simulink model "TST_BattU_VD"  (R2016b)
settings: Solver=FixedStepDiscrete  StartTime=0.0  StopTime=simTime  FixedStep=sampleTime  RelTol=1e-3
values from neighbouring files (symbols this model uses):
  testCase = 1    [initTST_BattU_VD_001.m]    (also in initTST_BattU_VD_002.m = 2; initTST_BattU_VD_003.m = 3; initTST_BattU_VD_004.m = 4; initTST_BattU_VD_005.m = 5)
libraries: simulink x21, UnitTest_Lib x15
settings Model: Creator=zhengjinyan  LastModifiedBy=zhengjinyan
settings DebuggingCC: SignalRangeChecking=error

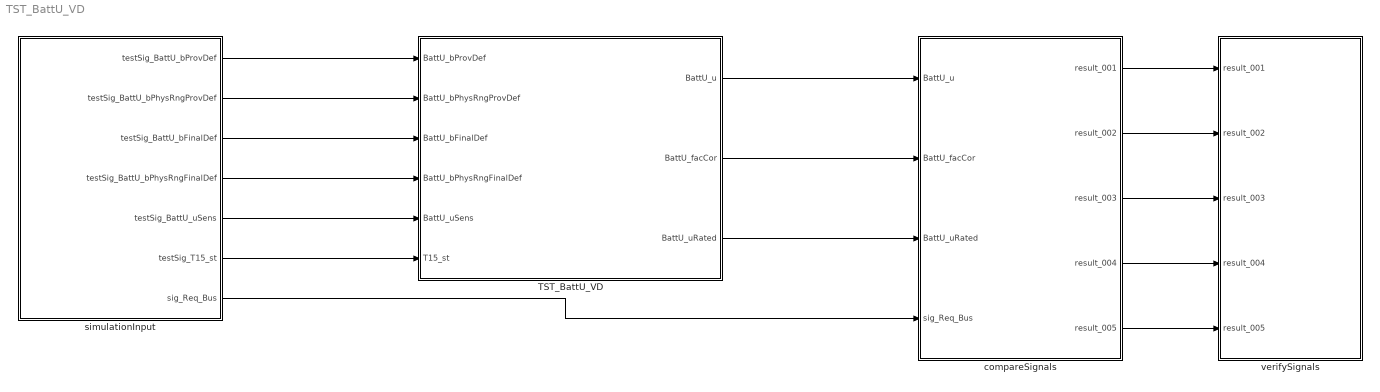
== system TST_BattU_VD ==
  TST_BattU_VD : Subsystem
  compareSignals : Subsystem
  simulationInput : Subsystem
  verifySignals : Subsystem
  wires:
  simulationInput/1(testSig_BattU_bProvDef) -> TST_BattU_VD/1(BattU_bProvDef)
  simulationInput/2(testSig_BattU_bPhysRngProvDef) -> TST_BattU_VD/2(BattU_bPhysRngProvDef)
  simulationInput/3(testSig_BattU_bFinalDef) -> TST_BattU_VD/3(BattU_bFinalDef)
  simulationInput/4(testSig_BattU_bPhysRngFinalDef) -> TST_BattU_VD/4(BattU_bPhysRngFinalDef)
  simulationInput/5(testSig_BattU_uSens) -> TST_BattU_VD/5(BattU_uSens)
  simulationInput/6(testSig_T15_st) -> TST_BattU_VD/6(T15_st)
  TST_BattU_VD/1(BattU_u) -> compareSignals/1(BattU_u)
  TST_BattU_VD/2(BattU_facCor) -> compareSignals/2(BattU_facCor)
  TST_BattU_VD/3(BattU_uRated) -> compareSignals/3(BattU_uRated)
  simulationInput/7(sig_Req_Bus) -> compareSignals/4(sig_Req_Bus)
  compareSignals/1(result_001) -> verifySignals/1(result_001)
  compareSignals/2(result_002) -> verifySignals/2(result_002)
  compareSignals/3(result_003) -> verifySignals/3(result_003)
  compareSignals/4(result_004) -> verifySignals/4(result_004)
  compareSignals/5(result_005) -> verifySignals/5(result_005)

== system TST_BattU_VD/TST_BattU_VD ==
  BattU_bProvDef : Inport
  BattU_bPhysRngProvDef : Inport  Port=2
  BattU_bFinalDef : Inport  Port=3
  BattU_bPhysRngFinalDef : Inport  Port=4
  BattU_uSens : Inport  Port=5
  T15_st : Inport  Port=6
  BattU_VD : ModelReference  ModelNameDialog=BattU_VD  SimulationMode=Normal  ModelReferenceVersion=1.13  TriggerPortName=function  TriggerPortTriggerType=function-call  TriggerPortStatesWhenEnabling=held
  Function_Call : simulink/Ports & Subsystems/Function-Call Generator  sample_time=sampleTime  numberOfIterations=1
  BattU_u : Outport
  BattU_facCor : Outport  Port=2
  BattU_uRated : Outport  Port=3
  wires:
  Function_Call/1 -> BattU_VD/Trigger
  BattU_bProvDef/1 -> BattU_VD/1
  BattU_bPhysRngProvDef/1 -> BattU_VD/2
  BattU_bFinalDef/1 -> BattU_VD/3
  BattU_bPhysRngFinalDef/1 -> BattU_VD/4
  BattU_uSens/1 -> BattU_VD/5
  T15_st/1 -> BattU_VD/6
  BattU_VD/1 -> BattU_u/1
  BattU_VD/2 -> BattU_facCor/1
  BattU_VD/3 -> BattU_uRated/1

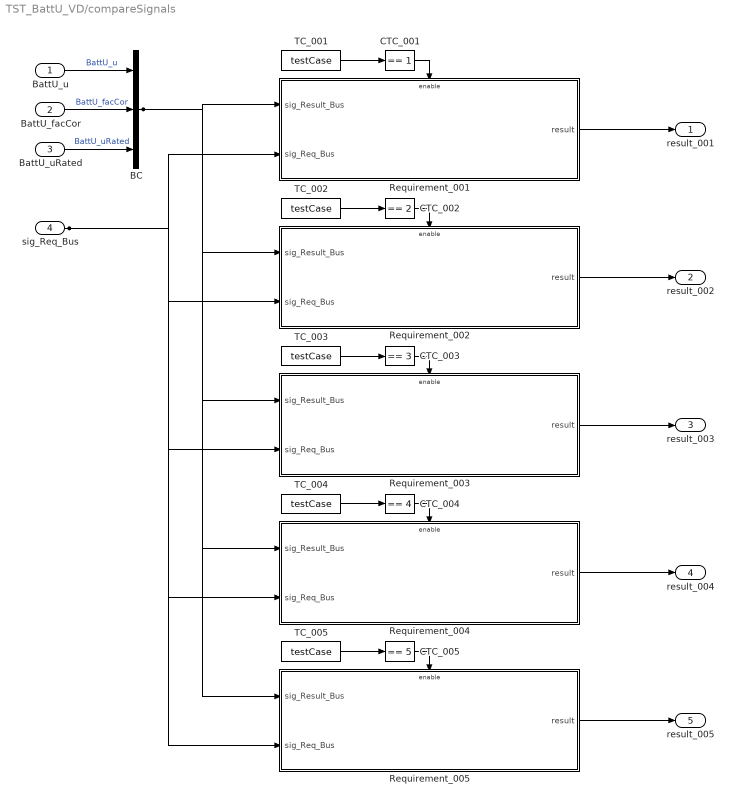
== system TST_BattU_VD/compareSignals ==
  BattU_u : Inport
  BattU_facCor : Inport  Port=2
  BattU_uRated : Inport  Port=3
  sig_Req_Bus : Inport  Port=4
  BC : BusCreator  Inputs=3
  CTC_001 : simulink/Logic and Bit Operations/Compare To Constant  relop===  const=1  OutDataTypeStr=boolean
  CTC_002 : simulink/Logic and Bit Operations/Compare To Constant  relop===  const=2  OutDataTypeStr=boolean
  CTC_003 : simulink/Logic and Bit Operations/Compare To Constant  relop===  const=3  OutDataTypeStr=boolean
  CTC_004 : simulink/Logic and Bit Operations/Compare To Constant  relop===  const=4  OutDataTypeStr=boolean
  CTC_005 : simulink/Logic and Bit Operations/Compare To Constant  relop===  const=5  OutDataTypeStr=boolean
  Requirement_001 : Subsystem
  Requirement_002 : Subsystem
  Requirement_003 : Subsystem
  Requirement_004 : Subsystem
  Requirement_005 : Subsystem
  TC_001 : Constant  Value=testCase
  TC_002 : Constant  Value=testCase
  TC_003 : Constant  Value=testCase
  TC_004 : Constant  Value=testCase
  TC_005 : Constant  Value=testCase
  result_001 : Outport
  result_002 : Outport  Port=2
  result_003 : Outport  Port=3
  result_004 : Outport  Port=4
  result_005 : Outport  Port=5
  wires:
  BattU_u/1 -> BC/1  "BattU_u"
  BattU_facCor/1 -> BC/2  "BattU_facCor"
  BattU_uRated/1 -> BC/3  "BattU_uRated"
  TC_001/1 -> CTC_001/1
  CTC_001/1 -> Requirement_001/Enable
  sig_Req_Bus/1 -> Requirement_001/2(sig_Req_Bus), Requirement_002/2(sig_Req_Bus), Requirement_003/2(sig_Req_Bus), Requirement_004/2(sig_Req_Bus), Requirement_005/2(sig_Req_Bus)
  BC/1 -> Requirement_001/1(sig_Result_Bus), Requirement_002/1(sig_Result_Bus), Requirement_003/1(sig_Result_Bus), Requirement_004/1(sig_Result_Bus), Requirement_005/1(sig_Result_Bus)
  Requirement_001/1(result) -> result_001/1
  TC_002/1 -> CTC_002/1
  CTC_002/1 -> Requirement_002/Enable
  Requirement_002/1(result) -> result_002/1
  TC_003/1 -> CTC_003/1
  CTC_003/1 -> Requirement_003/Enable
  Requirement_003/1(result) -> result_003/1
  TC_004/1 -> CTC_004/1
  CTC_004/1 -> Requirement_004/Enable
  Requirement_004/1(result) -> result_004/1
  TC_005/1 -> CTC_005/1
  CTC_005/1 -> Requirement_005/Enable
  Requirement_005/1(result) -> result_005/1

== system TST_BattU_VD/simulationInput ==
  BS : BusSelector  OutputSignals=testSig_BattU_bProvDef,testSig_BattU_bPhysRngProvDef,testSig_BattU_bFinalDef,testSig_BattU_bPhysRngFinalDef,testSig_BattU_uSens,testSig_T15_st
  MPSw : MultiPortSwitch  Inputs=5  SaturateOnIntegerOverflow=on  InputSameDT=on
  TestCase : Constant  Value=testCase
  testSignals_R001 : Subsystem
  testSignals_R002 : Subsystem
  testSignals_R003 : Subsystem
  testSignals_R004 : Subsystem
  testSignals_R005 : Subsystem
  testSig_BattU_bProvDef : Outport
  testSig_BattU_bPhysRngProvDef : Outport  Port=2
  testSig_BattU_bFinalDef : Outport  Port=3
  testSig_BattU_bPhysRngFinalDef : Outport  Port=4
  testSig_BattU_uSens : Outport  Port=5
  testSig_T15_st : Outport  Port=6
  sig_Req_Bus : Outport  Port=7
  wires:
  BS/1 -> testSig_BattU_bProvDef/1  "<testSig_BattU_bProvDef>"
  BS/2 -> testSig_BattU_bPhysRngProvDef/1  "<testSig_BattU_bPhysRngProvDef>"
  BS/3 -> testSig_BattU_bFinalDef/1  "<testSig_BattU_bFinalDef>"
  BS/4 -> testSig_BattU_bPhysRngFinalDef/1  "<testSig_BattU_bPhysRngFinalDef>"
  BS/5 -> testSig_BattU_uSens/1  "<testSig_BattU_uSens>"
  BS/6 -> testSig_T15_st/1  "<testSig_T15_st>"
  MPSw/1 -> BS/1, sig_Req_Bus/1
  TestCase/1 -> MPSw/1
  testSignals_R001/1(testSignals) -> MPSw/2
  testSignals_R002/1(testSignals) -> MPSw/3
  testSignals_R003/1(testSignals) -> MPSw/4
  testSignals_R004/1(testSignals) -> MPSw/5
  testSignals_R005/1(testSignals) -> MPSw/6

== system TST_BattU_VD/verifySignals ==
  result_001 : Inport
  result_002 : Inport  Port=2
  result_003 : Inport  Port=3
  result_004 : Inport  Port=4
  result_005 : Inport  Port=5
  Assertion_001 : Assertion  Enabled=off
  Assertion_002 : Assertion  Enabled=off
  Assertion_003 : Assertion  Enabled=off
  Assertion_004 : Assertion  Enabled=off
  Assertion_005 : Assertion  Enabled=off
  wires:
  result_001/1 -> Assertion_001/1
  result_002/1 -> Assertion_002/1
  result_003/1 -> Assertion_003/1
  result_004/1 -> Assertion_004/1
  result_005/1 -> Assertion_005/1

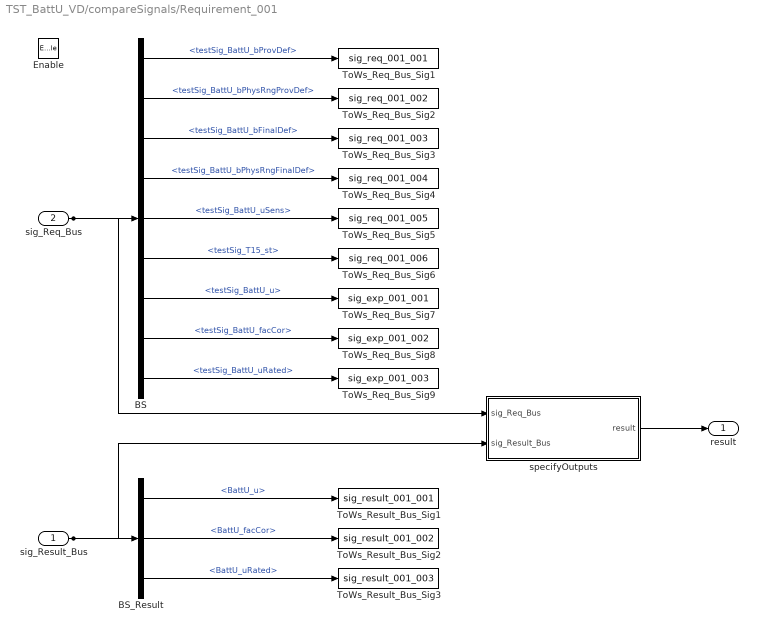
== system TST_BattU_VD/compareSignals/Requirement_001 ==
  sig_Result_Bus : Inport
  sig_Req_Bus : Inport  Port=2
  Enable : EnablePort
  BS : BusSelector  OutputSignals=testSig_BattU_bProvDef,testSig_BattU_bPhysRngProvDef,testSig_BattU_bFinalDef,testSig_BattU_bPhysRngFinalDef,testSig_BattU_uSens,testSig_T15_st,testSig_BattU_u,testSig_BattU_facCor,testSig_BattU_uRated
  BS_Result : BusSelector  OutputSignals=BattU_u,BattU_facCor,BattU_uRated
  ToWs_Req_Bus_Sig1 : ToWorkspace  VariableName=sig_req_001_001  SaveFormat=Structure With Time
  ToWs_Req_Bus_Sig2 : ToWorkspace  VariableName=sig_req_001_002  SaveFormat=Structure With Time
  ToWs_Req_Bus_Sig3 : ToWorkspace  VariableName=sig_req_001_003  SaveFormat=Structure With Time
  ToWs_Req_Bus_Sig4 : ToWorkspace  VariableName=sig_req_001_004  SaveFormat=Structure With Time
  ToWs_Req_Bus_Sig5 : ToWorkspace  VariableName=sig_req_001_005  SaveFormat=Structure With Time
  ToWs_Req_Bus_Sig6 : ToWorkspace  VariableName=sig_req_001_006  SaveFormat=Structure With Time
  ToWs_Req_Bus_Sig7 : ToWorkspace  VariableName=sig_exp_001_001  SaveFormat=Structure With Time
  ToWs_Req_Bus_Sig8 : ToWorkspace  VariableName=sig_exp_001_002  SaveFormat=Structure With Time
  ToWs_Req_Bus_Sig9 : ToWorkspace  VariableName=sig_exp_001_003  SaveFormat=Structure With Time
  ToWs_Result_Bus_Sig1 : ToWorkspace  VariableName=sig_result_001_001  SaveFormat=Structure With Time
  ToWs_Result_Bus_Sig2 : ToWorkspace  VariableName=sig_result_001_002  SaveFormat=Structure With Time
  ToWs_Result_Bus_Sig3 : ToWorkspace  VariableName=sig_result_001_003  SaveFormat=Structure With Time
  specifyOutputs : Subsystem
  result : Outport
  wires:
  sig_Req_Bus/1 -> BS/1, specifyOutputs/1(sig_Req_Bus)
  BS/1 -> ToWs_Req_Bus_Sig1/1  "<testSig_BattU_bProvDef>"
  BS/2 -> ToWs_Req_Bus_Sig2/1  "<testSig_BattU_bPhysRngProvDef>"
  BS/3 -> ToWs_Req_Bus_Sig3/1  "<testSig_BattU_bFinalDef>"
  BS/4 -> ToWs_Req_Bus_Sig4/1  "<testSig_BattU_bPhysRngFinalDef>"
  BS/5 -> ToWs_Req_Bus_Sig5/1  "<testSig_BattU_uSens>"
  BS/6 -> ToWs_Req_Bus_Sig6/1  "<testSig_T15_st>"
  BS/7 -> ToWs_Req_Bus_Sig7/1  "<testSig_BattU_u>"
  BS/8 -> ToWs_Req_Bus_Sig8/1  "<testSig_BattU_facCor>"
  BS/9 -> ToWs_Req_Bus_Sig9/1  "<testSig_BattU_uRated>"
  sig_Result_Bus/1 -> BS_Result/1, specifyOutputs/2(sig_Result_Bus)
  BS_Result/1 -> ToWs_Result_Bus_Sig1/1  "<BattU_u>"
  BS_Result/2 -> ToWs_Result_Bus_Sig2/1  "<BattU_facCor>"
  BS_Result/3 -> ToWs_Result_Bus_Sig3/1  "<BattU_uRated>"
  specifyOutputs/1(result) -> result/1

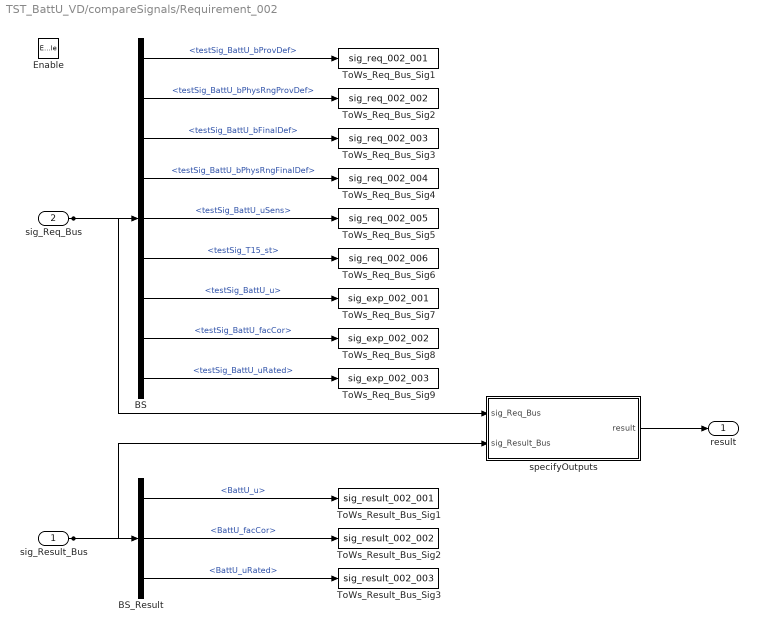
== system TST_BattU_VD/compareSignals/Requirement_002 ==
  sig_Result_Bus : Inport
  sig_Req_Bus : Inport  Port=2
  Enable : EnablePort
  BS : BusSelector  OutputSignals=testSig_BattU_bProvDef,testSig_BattU_bPhysRngProvDef,testSig_BattU_bFinalDef,testSig_BattU_bPhysRngFinalDef,testSig_BattU_uSens,testSig_T15_st,testSig_BattU_u,testSig_BattU_facCor,testSig_BattU_uRated
  BS_Result : BusSelector  OutputSignals=BattU_u,BattU_facCor,BattU_uRated
  ToWs_Req_Bus_Sig1 : ToWorkspace  VariableName=sig_req_002_001  SaveFormat=Structure With Time
  ToWs_Req_Bus_Sig2 : ToWorkspace  VariableName=sig_req_002_002  SaveFormat=Structure With Time
  ToWs_Req_Bus_Sig3 : ToWorkspace  VariableName=sig_req_002_003  SaveFormat=Structure With Time
  ToWs_Req_Bus_Sig4 : ToWorkspace  VariableName=sig_req_002_004  SaveFormat=Structure With Time
  ToWs_Req_Bus_Sig5 : ToWorkspace  VariableName=sig_req_002_005  SaveFormat=Structure With Time
  ToWs_Req_Bus_Sig6 : ToWorkspace  VariableName=sig_req_002_006  SaveFormat=Structure With Time
  ToWs_Req_Bus_Sig7 : ToWorkspace  VariableName=sig_exp_002_001  SaveFormat=Structure With Time
  ToWs_Req_Bus_Sig8 : ToWorkspace  VariableName=sig_exp_002_002  SaveFormat=Structure With Time
  ToWs_Req_Bus_Sig9 : ToWorkspace  VariableName=sig_exp_002_003  SaveFormat=Structure With Time
  ToWs_Result_Bus_Sig1 : ToWorkspace  VariableName=sig_result_002_001  SaveFormat=Structure With Time
  ToWs_Result_Bus_Sig2 : ToWorkspace  VariableName=sig_result_002_002  SaveFormat=Structure With Time
  ToWs_Result_Bus_Sig3 : ToWorkspace  VariableName=sig_result_002_003  SaveFormat=Structure With Time
  specifyOutputs : Subsystem
  result : Outport
  wires:
  sig_Req_Bus/1 -> BS/1, specifyOutputs/1(sig_Req_Bus)
  BS/1 -> ToWs_Req_Bus_Sig1/1  "<testSig_BattU_bProvDef>"
  BS/2 -> ToWs_Req_Bus_Sig2/1  "<testSig_BattU_bPhysRngProvDef>"
  BS/3 -> ToWs_Req_Bus_Sig3/1  "<testSig_BattU_bFinalDef>"
  BS/4 -> ToWs_Req_Bus_Sig4/1  "<testSig_BattU_bPhysRngFinalDef>"
  BS/5 -> ToWs_Req_Bus_Sig5/1  "<testSig_BattU_uSens>"
  BS/6 -> ToWs_Req_Bus_Sig6/1  "<testSig_T15_st>"
  BS/7 -> ToWs_Req_Bus_Sig7/1  "<testSig_BattU_u>"
  BS/8 -> ToWs_Req_Bus_Sig8/1  "<testSig_BattU_facCor>"
  BS/9 -> ToWs_Req_Bus_Sig9/1  "<testSig_BattU_uRated>"
  sig_Result_Bus/1 -> BS_Result/1, specifyOutputs/2(sig_Result_Bus)
  BS_Result/1 -> ToWs_Result_Bus_Sig1/1  "<BattU_u>"
  BS_Result/2 -> ToWs_Result_Bus_Sig2/1  "<BattU_facCor>"
  BS_Result/3 -> ToWs_Result_Bus_Sig3/1  "<BattU_uRated>"
  specifyOutputs/1(result) -> result/1

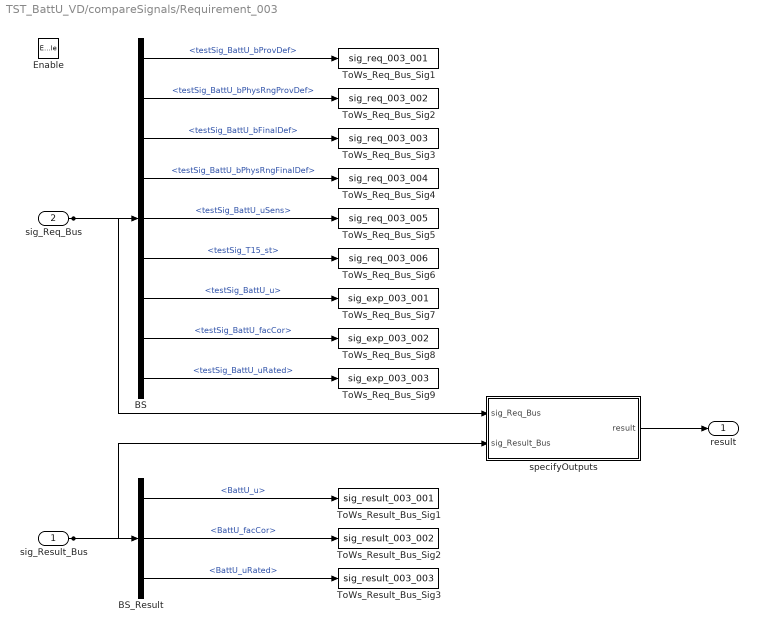
== system TST_BattU_VD/compareSignals/Requirement_003 ==
  sig_Result_Bus : Inport
  sig_Req_Bus : Inport  Port=2
  Enable : EnablePort
  BS : BusSelector  OutputSignals=testSig_BattU_bProvDef,testSig_BattU_bPhysRngProvDef,testSig_BattU_bFinalDef,testSig_BattU_bPhysRngFinalDef,testSig_BattU_uSens,testSig_T15_st,testSig_BattU_u,testSig_BattU_facCor,testSig_BattU_uRated
  BS_Result : BusSelector  OutputSignals=BattU_u,BattU_facCor,BattU_uRated
  ToWs_Req_Bus_Sig1 : ToWorkspace  VariableName=sig_req_003_001  SaveFormat=Structure With Time
  ToWs_Req_Bus_Sig2 : ToWorkspace  VariableName=sig_req_003_002  SaveFormat=Structure With Time
  ToWs_Req_Bus_Sig3 : ToWorkspace  VariableName=sig_req_003_003  SaveFormat=Structure With Time
  ToWs_Req_Bus_Sig4 : ToWorkspace  VariableName=sig_req_003_004  SaveFormat=Structure With Time
  ToWs_Req_Bus_Sig5 : ToWorkspace  VariableName=sig_req_003_005  SaveFormat=Structure With Time
  ToWs_Req_Bus_Sig6 : ToWorkspace  VariableName=sig_req_003_006  SaveFormat=Structure With Time
  ToWs_Req_Bus_Sig7 : ToWorkspace  VariableName=sig_exp_003_001  SaveFormat=Structure With Time
  ToWs_Req_Bus_Sig8 : ToWorkspace  VariableName=sig_exp_003_002  SaveFormat=Structure With Time
  ToWs_Req_Bus_Sig9 : ToWorkspace  VariableName=sig_exp_003_003  SaveFormat=Structure With Time
  ToWs_Result_Bus_Sig1 : ToWorkspace  VariableName=sig_result_003_001  SaveFormat=Structure With Time
  ToWs_Result_Bus_Sig2 : ToWorkspace  VariableName=sig_result_003_002  SaveFormat=Structure With Time
  ToWs_Result_Bus_Sig3 : ToWorkspace  VariableName=sig_result_003_003  SaveFormat=Structure With Time
  specifyOutputs : Subsystem
  result : Outport
  wires:
  sig_Req_Bus/1 -> BS/1, specifyOutputs/1(sig_Req_Bus)
  BS/1 -> ToWs_Req_Bus_Sig1/1  "<testSig_BattU_bProvDef>"
  BS/2 -> ToWs_Req_Bus_Sig2/1  "<testSig_BattU_bPhysRngProvDef>"
  BS/3 -> ToWs_Req_Bus_Sig3/1  "<testSig_BattU_bFinalDef>"
  BS/4 -> ToWs_Req_Bus_Sig4/1  "<testSig_BattU_bPhysRngFinalDef>"
  BS/5 -> ToWs_Req_Bus_Sig5/1  "<testSig_BattU_uSens>"
  BS/6 -> ToWs_Req_Bus_Sig6/1  "<testSig_T15_st>"
  BS/7 -> ToWs_Req_Bus_Sig7/1  "<testSig_BattU_u>"
  BS/8 -> ToWs_Req_Bus_Sig8/1  "<testSig_BattU_facCor>"
  BS/9 -> ToWs_Req_Bus_Sig9/1  "<testSig_BattU_uRated>"
  sig_Result_Bus/1 -> BS_Result/1, specifyOutputs/2(sig_Result_Bus)
  BS_Result/1 -> ToWs_Result_Bus_Sig1/1  "<BattU_u>"
  BS_Result/2 -> ToWs_Result_Bus_Sig2/1  "<BattU_facCor>"
  BS_Result/3 -> ToWs_Result_Bus_Sig3/1  "<BattU_uRated>"
  specifyOutputs/1(result) -> result/1

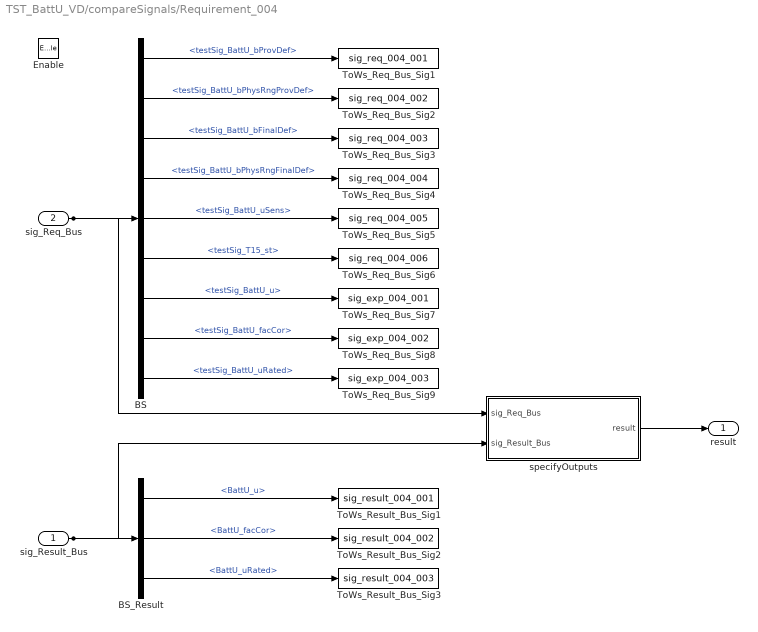
== system TST_BattU_VD/compareSignals/Requirement_004 ==
  sig_Result_Bus : Inport
  sig_Req_Bus : Inport  Port=2
  Enable : EnablePort
  BS : BusSelector  OutputSignals=testSig_BattU_bProvDef,testSig_BattU_bPhysRngProvDef,testSig_BattU_bFinalDef,testSig_BattU_bPhysRngFinalDef,testSig_BattU_uSens,testSig_T15_st,testSig_BattU_u,testSig_BattU_facCor,testSig_BattU_uRated
  BS_Result : BusSelector  OutputSignals=BattU_u,BattU_facCor,BattU_uRated
  ToWs_Req_Bus_Sig1 : ToWorkspace  VariableName=sig_req_004_001  SaveFormat=Structure With Time
  ToWs_Req_Bus_Sig2 : ToWorkspace  VariableName=sig_req_004_002  SaveFormat=Structure With Time
  ToWs_Req_Bus_Sig3 : ToWorkspace  VariableName=sig_req_004_003  SaveFormat=Structure With Time
  ToWs_Req_Bus_Sig4 : ToWorkspace  VariableName=sig_req_004_004  SaveFormat=Structure With Time
  ToWs_Req_Bus_Sig5 : ToWorkspace  VariableName=sig_req_004_005  SaveFormat=Structure With Time
  ToWs_Req_Bus_Sig6 : ToWorkspace  VariableName=sig_req_004_006  SaveFormat=Structure With Time
  ToWs_Req_Bus_Sig7 : ToWorkspace  VariableName=sig_exp_004_001  SaveFormat=Structure With Time
  ToWs_Req_Bus_Sig8 : ToWorkspace  VariableName=sig_exp_004_002  SaveFormat=Structure With Time
  ToWs_Req_Bus_Sig9 : ToWorkspace  VariableName=sig_exp_004_003  SaveFormat=Structure With Time
  ToWs_Result_Bus_Sig1 : ToWorkspace  VariableName=sig_result_004_001  SaveFormat=Structure With Time
  ToWs_Result_Bus_Sig2 : ToWorkspace  VariableName=sig_result_004_002  SaveFormat=Structure With Time
  ToWs_Result_Bus_Sig3 : ToWorkspace  VariableName=sig_result_004_003  SaveFormat=Structure With Time
  specifyOutputs : Subsystem
  result : Outport
  wires:
  sig_Req_Bus/1 -> BS/1, specifyOutputs/1(sig_Req_Bus)
  BS/1 -> ToWs_Req_Bus_Sig1/1  "<testSig_BattU_bProvDef>"
  BS/2 -> ToWs_Req_Bus_Sig2/1  "<testSig_BattU_bPhysRngProvDef>"
  BS/3 -> ToWs_Req_Bus_Sig3/1  "<testSig_BattU_bFinalDef>"
  BS/4 -> ToWs_Req_Bus_Sig4/1  "<testSig_BattU_bPhysRngFinalDef>"
  BS/5 -> ToWs_Req_Bus_Sig5/1  "<testSig_BattU_uSens>"
  BS/6 -> ToWs_Req_Bus_Sig6/1  "<testSig_T15_st>"
  BS/7 -> ToWs_Req_Bus_Sig7/1  "<testSig_BattU_u>"
  BS/8 -> ToWs_Req_Bus_Sig8/1  "<testSig_BattU_facCor>"
  BS/9 -> ToWs_Req_Bus_Sig9/1  "<testSig_BattU_uRated>"
  sig_Result_Bus/1 -> BS_Result/1, specifyOutputs/2(sig_Result_Bus)
  BS_Result/1 -> ToWs_Result_Bus_Sig1/1  "<BattU_u>"
  BS_Result/2 -> ToWs_Result_Bus_Sig2/1  "<BattU_facCor>"
  BS_Result/3 -> ToWs_Result_Bus_Sig3/1  "<BattU_uRated>"
  specifyOutputs/1(result) -> result/1

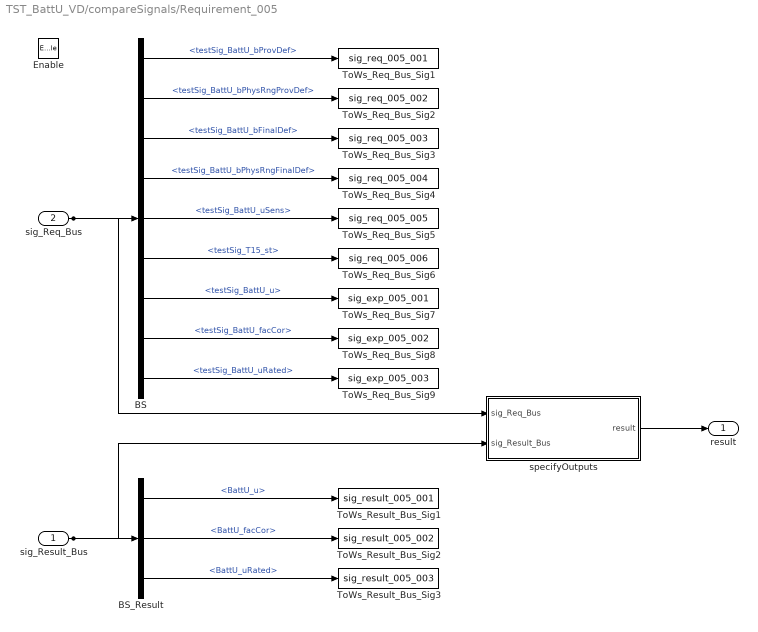
== system TST_BattU_VD/compareSignals/Requirement_005 ==
  sig_Result_Bus : Inport
  sig_Req_Bus : Inport  Port=2
  Enable : EnablePort
  BS : BusSelector  OutputSignals=testSig_BattU_bProvDef,testSig_BattU_bPhysRngProvDef,testSig_BattU_bFinalDef,testSig_BattU_bPhysRngFinalDef,testSig_BattU_uSens,testSig_T15_st,testSig_BattU_u,testSig_BattU_facCor,testSig_BattU_uRated
  BS_Result : BusSelector  OutputSignals=BattU_u,BattU_facCor,BattU_uRated
  ToWs_Req_Bus_Sig1 : ToWorkspace  VariableName=sig_req_005_001  SaveFormat=Structure With Time
  ToWs_Req_Bus_Sig2 : ToWorkspace  VariableName=sig_req_005_002  SaveFormat=Structure With Time
  ToWs_Req_Bus_Sig3 : ToWorkspace  VariableName=sig_req_005_003  SaveFormat=Structure With Time
  ToWs_Req_Bus_Sig4 : ToWorkspace  VariableName=sig_req_005_004  SaveFormat=Structure With Time
  ToWs_Req_Bus_Sig5 : ToWorkspace  VariableName=sig_req_005_005  SaveFormat=Structure With Time
  ToWs_Req_Bus_Sig6 : ToWorkspace  VariableName=sig_req_005_006  SaveFormat=Structure With Time
  ToWs_Req_Bus_Sig7 : ToWorkspace  VariableName=sig_exp_005_001  SaveFormat=Structure With Time
  ToWs_Req_Bus_Sig8 : ToWorkspace  VariableName=sig_exp_005_002  SaveFormat=Structure With Time
  ToWs_Req_Bus_Sig9 : ToWorkspace  VariableName=sig_exp_005_003  SaveFormat=Structure With Time
  ToWs_Result_Bus_Sig1 : ToWorkspace  VariableName=sig_result_005_001  SaveFormat=Structure With Time
  ToWs_Result_Bus_Sig2 : ToWorkspace  VariableName=sig_result_005_002  SaveFormat=Structure With Time
  ToWs_Result_Bus_Sig3 : ToWorkspace  VariableName=sig_result_005_003  SaveFormat=Structure With Time
  specifyOutputs : Subsystem
  result : Outport
  wires:
  sig_Req_Bus/1 -> BS/1, specifyOutputs/1(sig_Req_Bus)
  BS/1 -> ToWs_Req_Bus_Sig1/1  "<testSig_BattU_bProvDef>"
  BS/2 -> ToWs_Req_Bus_Sig2/1  "<testSig_BattU_bPhysRngProvDef>"
  BS/3 -> ToWs_Req_Bus_Sig3/1  "<testSig_BattU_bFinalDef>"
  BS/4 -> ToWs_Req_Bus_Sig4/1  "<testSig_BattU_bPhysRngFinalDef>"
  BS/5 -> ToWs_Req_Bus_Sig5/1  "<testSig_BattU_uSens>"
  BS/6 -> ToWs_Req_Bus_Sig6/1  "<testSig_T15_st>"
  BS/7 -> ToWs_Req_Bus_Sig7/1  "<testSig_BattU_u>"
  BS/8 -> ToWs_Req_Bus_Sig8/1  "<testSig_BattU_facCor>"
  BS/9 -> ToWs_Req_Bus_Sig9/1  "<testSig_BattU_uRated>"
  sig_Result_Bus/1 -> BS_Result/1, specifyOutputs/2(sig_Result_Bus)
  BS_Result/1 -> ToWs_Result_Bus_Sig1/1  "<BattU_u>"
  BS_Result/2 -> ToWs_Result_Bus_Sig2/1  "<BattU_facCor>"
  BS_Result/3 -> ToWs_Result_Bus_Sig3/1  "<BattU_uRated>"
  specifyOutputs/1(result) -> result/1

== system TST_BattU_VD/simulationInput/testSignals_R001 ==
  BC : BusCreator  Inputs=9
  spec_BattU_bFinalDef : FromWorkspace  VariableName=testSig_BattU_bFinalDef  Interpolate=off  OutputAfterFinalValue=Holding final value
  spec_BattU_bPhysRngFinalDef : FromWorkspace  VariableName=testSig_BattU_bPhysRngFinalDef  Interpolate=off  OutputAfterFinalValue=Holding final value
  spec_BattU_bPhysRngProvDef : FromWorkspace  VariableName=testSig_BattU_bPhysRngProvDef  Interpolate=off  OutputAfterFinalValue=Holding final value
  spec_BattU_bProvDef : FromWorkspace  VariableName=testSig_BattU_bProvDef  Interpolate=off  OutputAfterFinalValue=Holding final value
  spec_BattU_facCor : FromWorkspace  VariableName=testSig_BattU_facCor  Interpolate=off  OutputAfterFinalValue=Holding final value
  spec_BattU_u : FromWorkspace  VariableName=testSig_BattU_u  Interpolate=off  OutputAfterFinalValue=Holding final value
  spec_BattU_uRated : FromWorkspace  VariableName=testSig_BattU_uRated  Interpolate=off  OutputAfterFinalValue=Holding final value
  spec_BattU_uSens : FromWorkspace  VariableName=testSig_BattU_uSens  Interpolate=off  OutputAfterFinalValue=Holding final value
  spec_T15_st : FromWorkspace  VariableName=testSig_T15_st  Interpolate=off  OutputAfterFinalValue=Holding final value
  testSignals : Outport
  wires:
  BC/1 -> testSignals/1
  spec_BattU_bProvDef/1 -> BC/1  "testSig_BattU_bProvDef"
  spec_BattU_bPhysRngProvDef/1 -> BC/2  "testSig_BattU_bPhysRngProvDef"
  spec_BattU_bFinalDef/1 -> BC/3  "testSig_BattU_bFinalDef"
  spec_BattU_bPhysRngFinalDef/1 -> BC/4  "testSig_BattU_bPhysRngFinalDef"
  spec_BattU_uSens/1 -> BC/5  "testSig_BattU_uSens"
  spec_T15_st/1 -> BC/6  "testSig_T15_st"
  spec_BattU_u/1 -> BC/7  "testSig_BattU_u"
  spec_BattU_facCor/1 -> BC/8  "testSig_BattU_facCor"
  spec_BattU_uRated/1 -> BC/9  "testSig_BattU_uRated"

== system TST_BattU_VD/simulationInput/testSignals_R002 ==
  BC : BusCreator  Inputs=9
  spec_BattU_bFinalDef : FromWorkspace  VariableName=testSig_BattU_bFinalDef  Interpolate=off  OutputAfterFinalValue=Holding final value
  spec_BattU_bPhysRngFinalDef : FromWorkspace  VariableName=testSig_BattU_bPhysRngFinalDef  Interpolate=off  OutputAfterFinalValue=Holding final value
  spec_BattU_bPhysRngProvDef : FromWorkspace  VariableName=testSig_BattU_bPhysRngProvDef  Interpolate=off  OutputAfterFinalValue=Holding final value
  spec_BattU_bProvDef : FromWorkspace  VariableName=testSig_BattU_bProvDef  Interpolate=off  OutputAfterFinalValue=Holding final value
  spec_BattU_facCor : FromWorkspace  VariableName=testSig_BattU_facCor  Interpolate=off  OutputAfterFinalValue=Holding final value
  spec_BattU_u : FromWorkspace  VariableName=testSig_BattU_u  Interpolate=off  OutputAfterFinalValue=Holding final value
  spec_BattU_uRated : FromWorkspace  VariableName=testSig_BattU_uRated  Interpolate=off  OutputAfterFinalValue=Holding final value
  spec_BattU_uSens : FromWorkspace  VariableName=testSig_BattU_uSens  Interpolate=off  OutputAfterFinalValue=Holding final value
  spec_T15_st : FromWorkspace  VariableName=testSig_T15_st  Interpolate=off  OutputAfterFinalValue=Holding final value
  testSignals : Outport
  wires:
  BC/1 -> testSignals/1
  spec_BattU_bProvDef/1 -> BC/1  "testSig_BattU_bProvDef"
  spec_BattU_bPhysRngProvDef/1 -> BC/2  "testSig_BattU_bPhysRngProvDef"
  spec_BattU_bFinalDef/1 -> BC/3  "testSig_BattU_bFinalDef"
  spec_BattU_bPhysRngFinalDef/1 -> BC/4  "testSig_BattU_bPhysRngFinalDef"
  spec_BattU_uSens/1 -> BC/5  "testSig_BattU_uSens"
  spec_T15_st/1 -> BC/6  "testSig_T15_st"
  spec_BattU_u/1 -> BC/7  "testSig_BattU_u"
  spec_BattU_facCor/1 -> BC/8  "testSig_BattU_facCor"
  spec_BattU_uRated/1 -> BC/9  "testSig_BattU_uRated"

== system TST_BattU_VD/simulationInput/testSignals_R003 ==
  BC : BusCreator  Inputs=9
  spec_BattU_bFinalDef : FromWorkspace  VariableName=testSig_BattU_bFinalDef  Interpolate=off  OutputAfterFinalValue=Holding final value
  spec_BattU_bPhysRngFinalDef : FromWorkspace  VariableName=testSig_BattU_bPhysRngFinalDef  Interpolate=off  OutputAfterFinalValue=Holding final value
  spec_BattU_bPhysRngProvDef : FromWorkspace  VariableName=testSig_BattU_bPhysRngProvDef  Interpolate=off  OutputAfterFinalValue=Holding final value
  spec_BattU_bProvDef : FromWorkspace  VariableName=testSig_BattU_bProvDef  Interpolate=off  OutputAfterFinalValue=Holding final value
  spec_BattU_facCor : FromWorkspace  VariableName=testSig_BattU_facCor  Interpolate=off  OutputAfterFinalValue=Holding final value
  spec_BattU_u : FromWorkspace  VariableName=testSig_BattU_u  Interpolate=off  OutputAfterFinalValue=Holding final value
  spec_BattU_uRated : FromWorkspace  VariableName=testSig_BattU_uRated  Interpolate=off  OutputAfterFinalValue=Holding final value
  spec_BattU_uSens : FromWorkspace  VariableName=testSig_BattU_uSens  Interpolate=off  OutputAfterFinalValue=Holding final value
  spec_T15_st : FromWorkspace  VariableName=testSig_T15_st  Interpolate=off  OutputAfterFinalValue=Holding final value
  testSignals : Outport
  wires:
  BC/1 -> testSignals/1
  spec_BattU_bProvDef/1 -> BC/1  "testSig_BattU_bProvDef"
  spec_BattU_bPhysRngProvDef/1 -> BC/2  "testSig_BattU_bPhysRngProvDef"
  spec_BattU_bFinalDef/1 -> BC/3  "testSig_BattU_bFinalDef"
  spec_BattU_bPhysRngFinalDef/1 -> BC/4  "testSig_BattU_bPhysRngFinalDef"
  spec_BattU_uSens/1 -> BC/5  "testSig_BattU_uSens"
  spec_T15_st/1 -> BC/6  "testSig_T15_st"
  spec_BattU_u/1 -> BC/7  "testSig_BattU_u"
  spec_BattU_facCor/1 -> BC/8  "testSig_BattU_facCor"
  spec_BattU_uRated/1 -> BC/9  "testSig_BattU_uRated"

== system TST_BattU_VD/simulationInput/testSignals_R004 ==
  BC : BusCreator  Inputs=9
  spec_BattU_bFinalDef : FromWorkspace  VariableName=testSig_BattU_bFinalDef  Interpolate=off  OutputAfterFinalValue=Holding final value
  spec_BattU_bPhysRngFinalDef : FromWorkspace  VariableName=testSig_BattU_bPhysRngFinalDef  Interpolate=off  OutputAfterFinalValue=Holding final value
  spec_BattU_bPhysRngProvDef : FromWorkspace  VariableName=testSig_BattU_bPhysRngProvDef  Interpolate=off  OutputAfterFinalValue=Holding final value
  spec_BattU_bProvDef : FromWorkspace  VariableName=testSig_BattU_bProvDef  Interpolate=off  OutputAfterFinalValue=Holding final value
  spec_BattU_facCor : FromWorkspace  VariableName=testSig_BattU_facCor  Interpolate=off  OutputAfterFinalValue=Holding final value
  spec_BattU_u : FromWorkspace  VariableName=testSig_BattU_u  Interpolate=off  OutputAfterFinalValue=Holding final value
  spec_BattU_uRated : FromWorkspace  VariableName=testSig_BattU_uRated  Interpolate=off  OutputAfterFinalValue=Holding final value
  spec_BattU_uSens : FromWorkspace  VariableName=testSig_BattU_uSens  Interpolate=off  OutputAfterFinalValue=Holding final value
  spec_T15_st : FromWorkspace  VariableName=testSig_T15_st  Interpolate=off  OutputAfterFinalValue=Holding final value
  testSignals : Outport
  wires:
  BC/1 -> testSignals/1
  spec_BattU_bProvDef/1 -> BC/1  "testSig_BattU_bProvDef"
  spec_BattU_bPhysRngProvDef/1 -> BC/2  "testSig_BattU_bPhysRngProvDef"
  spec_BattU_bFinalDef/1 -> BC/3  "testSig_BattU_bFinalDef"
  spec_BattU_bPhysRngFinalDef/1 -> BC/4  "testSig_BattU_bPhysRngFinalDef"
  spec_BattU_uSens/1 -> BC/5  "testSig_BattU_uSens"
  spec_T15_st/1 -> BC/6  "testSig_T15_st"
  spec_BattU_u/1 -> BC/7  "testSig_BattU_u"
  spec_BattU_facCor/1 -> BC/8  "testSig_BattU_facCor"
  spec_BattU_uRated/1 -> BC/9  "testSig_BattU_uRated"

== system TST_BattU_VD/simulationInput/testSignals_R005 ==
  BC : BusCreator  Inputs=9
  spec_BattU_bFinalDef : FromWorkspace  VariableName=testSig_BattU_bFinalDef  Interpolate=off  OutputAfterFinalValue=Holding final value
  spec_BattU_bPhysRngFinalDef : FromWorkspace  VariableName=testSig_BattU_bPhysRngFinalDef  Interpolate=off  OutputAfterFinalValue=Holding final value
  spec_BattU_bPhysRngProvDef : FromWorkspace  VariableName=testSig_BattU_bPhysRngProvDef  Interpolate=off  OutputAfterFinalValue=Holding final value
  spec_BattU_bProvDef : FromWorkspace  VariableName=testSig_BattU_bProvDef  Interpolate=off  OutputAfterFinalValue=Holding final value
  spec_BattU_facCor : FromWorkspace  VariableName=testSig_BattU_facCor  Interpolate=off  OutputAfterFinalValue=Holding final value
  spec_BattU_u : FromWorkspace  VariableName=testSig_BattU_u  Interpolate=off  OutputAfterFinalValue=Holding final value
  spec_BattU_uRated : FromWorkspace  VariableName=testSig_BattU_uRated  Interpolate=off  OutputAfterFinalValue=Holding final value
  spec_BattU_uSens : FromWorkspace  VariableName=testSig_BattU_uSens  Interpolate=off  OutputAfterFinalValue=Holding final value
  spec_T15_st : FromWorkspace  VariableName=testSig_T15_st  Interpolate=off  OutputAfterFinalValue=Holding final value
  testSignals : Outport
  wires:
  BC/1 -> testSignals/1
  spec_BattU_bProvDef/1 -> BC/1  "testSig_BattU_bProvDef"
  spec_BattU_bPhysRngProvDef/1 -> BC/2  "testSig_BattU_bPhysRngProvDef"
  spec_BattU_bFinalDef/1 -> BC/3  "testSig_BattU_bFinalDef"
  spec_BattU_bPhysRngFinalDef/1 -> BC/4  "testSig_BattU_bPhysRngFinalDef"
  spec_BattU_uSens/1 -> BC/5  "testSig_BattU_uSens"
  spec_T15_st/1 -> BC/6  "testSig_T15_st"
  spec_BattU_u/1 -> BC/7  "testSig_BattU_u"
  spec_BattU_facCor/1 -> BC/8  "testSig_BattU_facCor"
  spec_BattU_uRated/1 -> BC/9  "testSig_BattU_uRated"

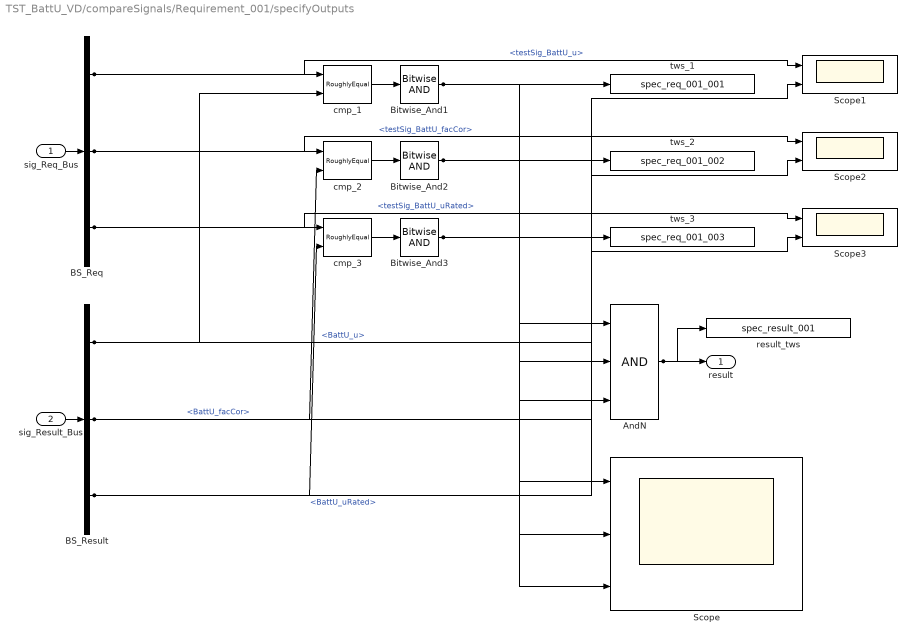
== system TST_BattU_VD/compareSignals/Requirement_001/specifyOutputs ==
  sig_Req_Bus : Inport
  sig_Result_Bus : Inport  Port=2
  AndN : Logic  Inputs=3
  BS_Req : BusSelector  OutputSignals=testSig_BattU_u,testSig_BattU_facCor,testSig_BattU_uRated
  BS_Result : BusSelector  OutputSignals=BattU_u,BattU_facCor,BattU_uRated
  Bitwise_And1 : simulink/Logic and Bit Operations/Bitwise Operator  logicop=AND  UseBitMask=off  BitMask=bin2dec('11011001')  BitMaskRealWorld=Stored Integer
  Bitwise_And2 : simulink/Logic and Bit Operations/Bitwise Operator  logicop=AND  UseBitMask=off  BitMask=bin2dec('11011001')  BitMaskRealWorld=Stored Integer
  Bitwise_And3 : simulink/Logic and Bit Operations/Bitwise Operator  logicop=AND  UseBitMask=off  BitMask=bin2dec('11011001')  BitMaskRealWorld=Stored Integer
  Scope : Scope  NumInputPorts=3
  Scope1 : Scope  NumInputPorts=2
  Scope2 : Scope  NumInputPorts=2
  Scope3 : Scope  NumInputPorts=2
  cmp_1 : UnitTest_Lib/RoughlyEqual  slope=0.1
  cmp_2 : UnitTest_Lib/RoughlyEqual  slope=0.1
  cmp_3 : UnitTest_Lib/RoughlyEqual  slope=0.1
  result_tws : ToWorkspace  VariableName=spec_result_001
  tws_1 : ToWorkspace  VariableName=spec_req_001_001
  tws_2 : ToWorkspace  VariableName=spec_req_001_002
  tws_3 : ToWorkspace  VariableName=spec_req_001_003
  result : Outport
  wires:
  sig_Req_Bus/1 -> BS_Req/1
  sig_Result_Bus/1 -> BS_Result/1
  AndN/1 -> result/1, result_tws/1
  BS_Req/1 -> cmp_1/1, Scope1/1  "<testSig_BattU_u>"
  BS_Result/1 -> cmp_1/2, Scope1/2  "<BattU_u>"
  cmp_1/1 -> Bitwise_And1/1
  Bitwise_And1/1 -> tws_1/1, AndN/1, Scope/1
  BS_Req/2 -> cmp_2/1, Scope2/1  "<testSig_BattU_facCor>"
  BS_Result/2 -> cmp_2/2, Scope2/2  "<BattU_facCor>"
  cmp_2/1 -> Bitwise_And2/1
  Bitwise_And2/1 -> tws_2/1, AndN/2, Scope/2
  BS_Req/3 -> cmp_3/1, Scope3/1  "<testSig_BattU_uRated>"
  BS_Result/3 -> cmp_3/2, Scope3/2  "<BattU_uRated>"
  cmp_3/1 -> Bitwise_And3/1
  Bitwise_And3/1 -> tws_3/1, AndN/3, Scope/3

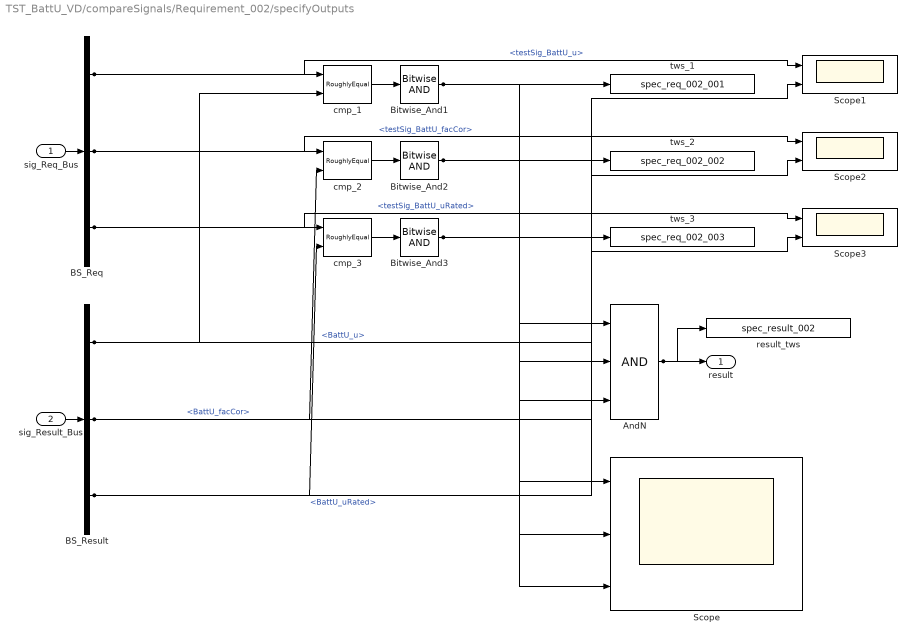
== system TST_BattU_VD/compareSignals/Requirement_002/specifyOutputs ==
  sig_Req_Bus : Inport
  sig_Result_Bus : Inport  Port=2
  AndN : Logic  Inputs=3
  BS_Req : BusSelector  OutputSignals=testSig_BattU_u,testSig_BattU_facCor,testSig_BattU_uRated
  BS_Result : BusSelector  OutputSignals=BattU_u,BattU_facCor,BattU_uRated
  Bitwise_And1 : simulink/Logic and Bit Operations/Bitwise Operator  logicop=AND  UseBitMask=off  BitMask=bin2dec('11011001')  BitMaskRealWorld=Stored Integer
  Bitwise_And2 : simulink/Logic and Bit Operations/Bitwise Operator  logicop=AND  UseBitMask=off  BitMask=bin2dec('11011001')  BitMaskRealWorld=Stored Integer
  Bitwise_And3 : simulink/Logic and Bit Operations/Bitwise Operator  logicop=AND  UseBitMask=off  BitMask=bin2dec('11011001')  BitMaskRealWorld=Stored Integer
  Scope : Scope  NumInputPorts=3
  Scope1 : Scope  NumInputPorts=2
  Scope2 : Scope  NumInputPorts=2
  Scope3 : Scope  NumInputPorts=2
  cmp_1 : UnitTest_Lib/RoughlyEqual  slope=0.1
  cmp_2 : UnitTest_Lib/RoughlyEqual  slope=0.1
  cmp_3 : UnitTest_Lib/RoughlyEqual  slope=0.1
  result_tws : ToWorkspace  VariableName=spec_result_002
  tws_1 : ToWorkspace  VariableName=spec_req_002_001
  tws_2 : ToWorkspace  VariableName=spec_req_002_002
  tws_3 : ToWorkspace  VariableName=spec_req_002_003
  result : Outport
  wires:
  sig_Req_Bus/1 -> BS_Req/1
  sig_Result_Bus/1 -> BS_Result/1
  AndN/1 -> result/1, result_tws/1
  BS_Req/1 -> cmp_1/1, Scope1/1  "<testSig_BattU_u>"
  BS_Result/1 -> cmp_1/2, Scope1/2  "<BattU_u>"
  cmp_1/1 -> Bitwise_And1/1
  Bitwise_And1/1 -> tws_1/1, AndN/1, Scope/1
  BS_Req/2 -> cmp_2/1, Scope2/1  "<testSig_BattU_facCor>"
  BS_Result/2 -> cmp_2/2, Scope2/2  "<BattU_facCor>"
  cmp_2/1 -> Bitwise_And2/1
  Bitwise_And2/1 -> tws_2/1, AndN/2, Scope/2
  BS_Req/3 -> cmp_3/1, Scope3/1  "<testSig_BattU_uRated>"
  BS_Result/3 -> cmp_3/2, Scope3/2  "<BattU_uRated>"
  cmp_3/1 -> Bitwise_And3/1
  Bitwise_And3/1 -> tws_3/1, AndN/3, Scope/3

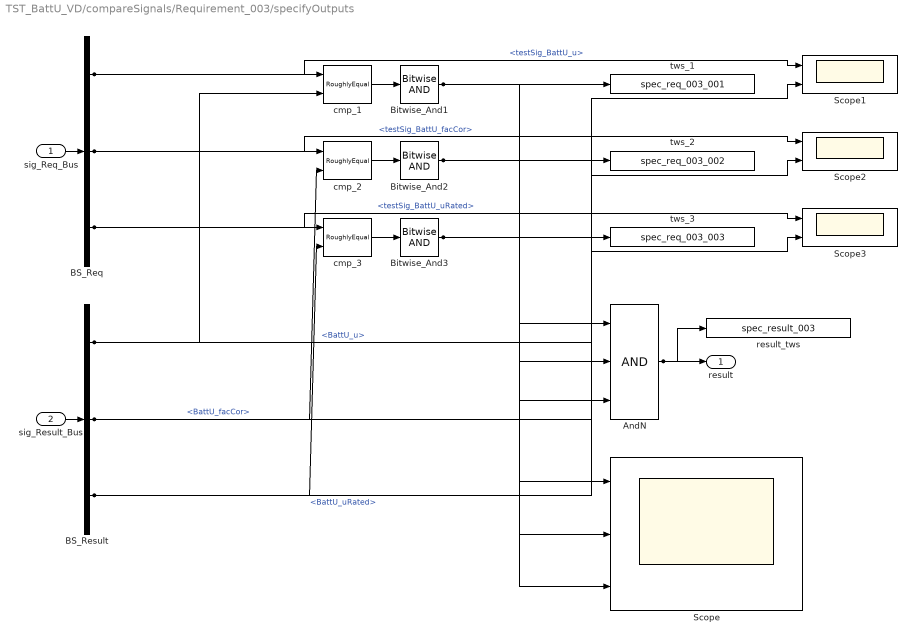
== system TST_BattU_VD/compareSignals/Requirement_003/specifyOutputs ==
  sig_Req_Bus : Inport
  sig_Result_Bus : Inport  Port=2
  AndN : Logic  Inputs=3
  BS_Req : BusSelector  OutputSignals=testSig_BattU_u,testSig_BattU_facCor,testSig_BattU_uRated
  BS_Result : BusSelector  OutputSignals=BattU_u,BattU_facCor,BattU_uRated
  Bitwise_And1 : simulink/Logic and Bit Operations/Bitwise Operator  logicop=AND  UseBitMask=off  BitMask=bin2dec('11011001')  BitMaskRealWorld=Stored Integer
  Bitwise_And2 : simulink/Logic and Bit Operations/Bitwise Operator  logicop=AND  UseBitMask=off  BitMask=bin2dec('11011001')  BitMaskRealWorld=Stored Integer
  Bitwise_And3 : simulink/Logic and Bit Operations/Bitwise Operator  logicop=AND  UseBitMask=off  BitMask=bin2dec('11011001')  BitMaskRealWorld=Stored Integer
  Scope : Scope  NumInputPorts=3
  Scope1 : Scope  NumInputPorts=2
  Scope2 : Scope  NumInputPorts=2
  Scope3 : Scope  NumInputPorts=2
  cmp_1 : UnitTest_Lib/RoughlyEqual  slope=0.1
  cmp_2 : UnitTest_Lib/RoughlyEqual  slope=0.1
  cmp_3 : UnitTest_Lib/RoughlyEqual  slope=0.1
  result_tws : ToWorkspace  VariableName=spec_result_003
  tws_1 : ToWorkspace  VariableName=spec_req_003_001
  tws_2 : ToWorkspace  VariableName=spec_req_003_002
  tws_3 : ToWorkspace  VariableName=spec_req_003_003
  result : Outport
  wires:
  sig_Req_Bus/1 -> BS_Req/1
  sig_Result_Bus/1 -> BS_Result/1
  AndN/1 -> result/1, result_tws/1
  BS_Req/1 -> cmp_1/1, Scope1/1  "<testSig_BattU_u>"
  BS_Result/1 -> cmp_1/2, Scope1/2  "<BattU_u>"
  cmp_1/1 -> Bitwise_And1/1
  Bitwise_And1/1 -> tws_1/1, AndN/1, Scope/1
  BS_Req/2 -> cmp_2/1, Scope2/1  "<testSig_BattU_facCor>"
  BS_Result/2 -> cmp_2/2, Scope2/2  "<BattU_facCor>"
  cmp_2/1 -> Bitwise_And2/1
  Bitwise_And2/1 -> tws_2/1, AndN/2, Scope/2
  BS_Req/3 -> cmp_3/1, Scope3/1  "<testSig_BattU_uRated>"
  BS_Result/3 -> cmp_3/2, Scope3/2  "<BattU_uRated>"
  cmp_3/1 -> Bitwise_And3/1
  Bitwise_And3/1 -> tws_3/1, AndN/3, Scope/3

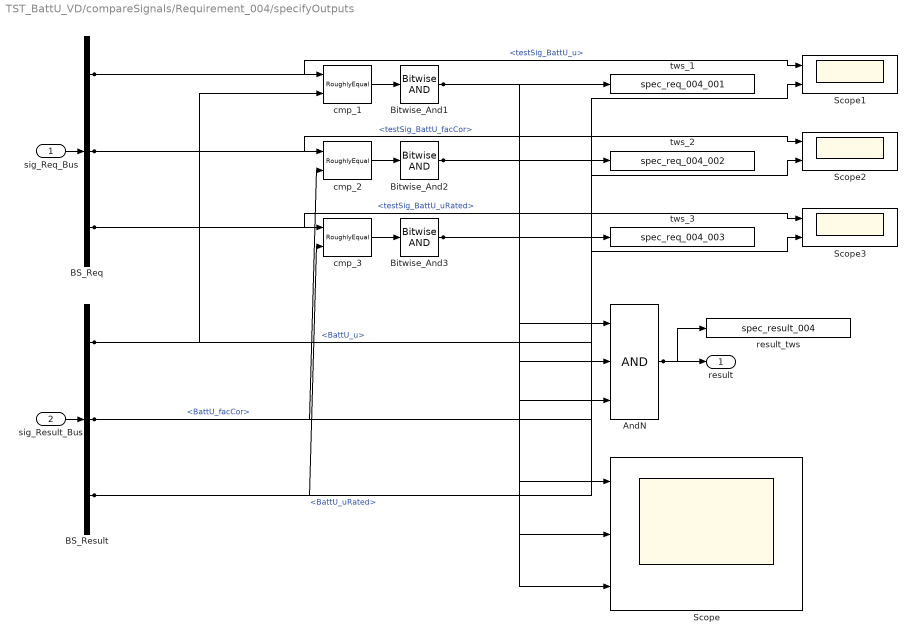
== system TST_BattU_VD/compareSignals/Requirement_004/specifyOutputs ==
  sig_Req_Bus : Inport
  sig_Result_Bus : Inport  Port=2
  AndN : Logic  Inputs=3
  BS_Req : BusSelector  OutputSignals=testSig_BattU_u,testSig_BattU_facCor,testSig_BattU_uRated
  BS_Result : BusSelector  OutputSignals=BattU_u,BattU_facCor,BattU_uRated
  Bitwise_And1 : simulink/Logic and Bit Operations/Bitwise Operator  logicop=AND  UseBitMask=off  BitMask=bin2dec('11011001')  BitMaskRealWorld=Stored Integer
  Bitwise_And2 : simulink/Logic and Bit Operations/Bitwise Operator  logicop=AND  UseBitMask=off  BitMask=bin2dec('11011001')  BitMaskRealWorld=Stored Integer
  Bitwise_And3 : simulink/Logic and Bit Operations/Bitwise Operator  logicop=AND  UseBitMask=off  BitMask=bin2dec('11011001')  BitMaskRealWorld=Stored Integer
  Scope : Scope  NumInputPorts=3
  Scope1 : Scope  NumInputPorts=2
  Scope2 : Scope  NumInputPorts=2
  Scope3 : Scope  NumInputPorts=2
  cmp_1 : UnitTest_Lib/RoughlyEqual  slope=0.1
  cmp_2 : UnitTest_Lib/RoughlyEqual  slope=0.1
  cmp_3 : UnitTest_Lib/RoughlyEqual  slope=0.1
  result_tws : ToWorkspace  VariableName=spec_result_004
  tws_1 : ToWorkspace  VariableName=spec_req_004_001
  tws_2 : ToWorkspace  VariableName=spec_req_004_002
  tws_3 : ToWorkspace  VariableName=spec_req_004_003
  result : Outport
  wires:
  sig_Req_Bus/1 -> BS_Req/1
  sig_Result_Bus/1 -> BS_Result/1
  AndN/1 -> result/1, result_tws/1
  BS_Req/1 -> cmp_1/1, Scope1/1  "<testSig_BattU_u>"
  BS_Result/1 -> cmp_1/2, Scope1/2  "<BattU_u>"
  cmp_1/1 -> Bitwise_And1/1
  Bitwise_And1/1 -> tws_1/1, AndN/1, Scope/1
  BS_Req/2 -> cmp_2/1, Scope2/1  "<testSig_BattU_facCor>"
  BS_Result/2 -> cmp_2/2, Scope2/2  "<BattU_facCor>"
  cmp_2/1 -> Bitwise_And2/1
  Bitwise_And2/1 -> tws_2/1, AndN/2, Scope/2
  BS_Req/3 -> cmp_3/1, Scope3/1  "<testSig_BattU_uRated>"
  BS_Result/3 -> cmp_3/2, Scope3/2  "<BattU_uRated>"
  cmp_3/1 -> Bitwise_And3/1
  Bitwise_And3/1 -> tws_3/1, AndN/3, Scope/3

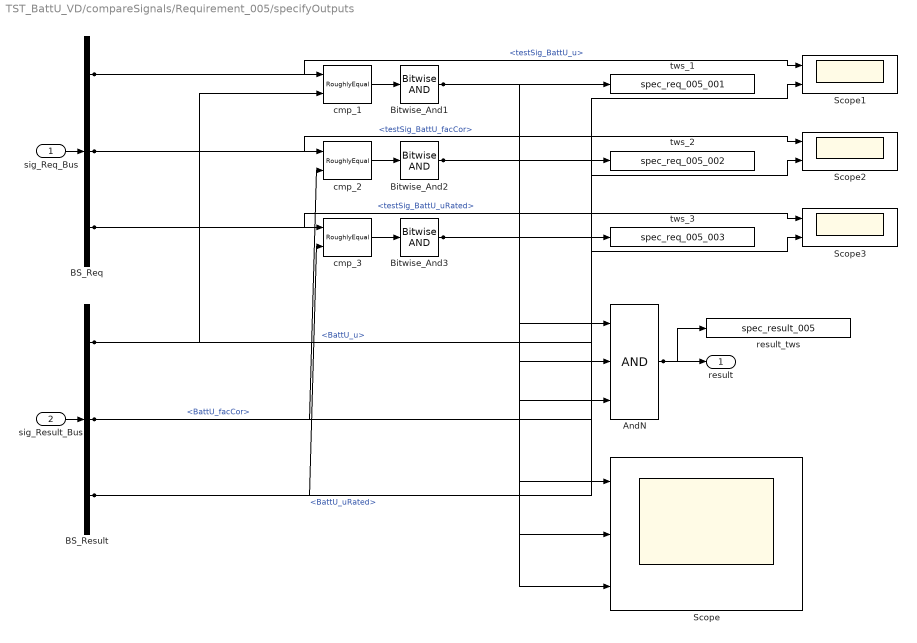
== system TST_BattU_VD/compareSignals/Requirement_005/specifyOutputs ==
  sig_Req_Bus : Inport
  sig_Result_Bus : Inport  Port=2
  AndN : Logic  Inputs=3
  BS_Req : BusSelector  OutputSignals=testSig_BattU_u,testSig_BattU_facCor,testSig_BattU_uRated
  BS_Result : BusSelector  OutputSignals=BattU_u,BattU_facCor,BattU_uRated
  Bitwise_And1 : simulink/Logic and Bit Operations/Bitwise Operator  logicop=AND  UseBitMask=off  BitMask=bin2dec('11011001')  BitMaskRealWorld=Stored Integer
  Bitwise_And2 : simulink/Logic and Bit Operations/Bitwise Operator  logicop=AND  UseBitMask=off  BitMask=bin2dec('11011001')  BitMaskRealWorld=Stored Integer
  Bitwise_And3 : simulink/Logic and Bit Operations/Bitwise Operator  logicop=AND  UseBitMask=off  BitMask=bin2dec('11011001')  BitMaskRealWorld=Stored Integer
  Scope : Scope  NumInputPorts=3
  Scope1 : Scope  NumInputPorts=2
  Scope2 : Scope  NumInputPorts=2
  Scope3 : Scope  NumInputPorts=2
  cmp_1 : UnitTest_Lib/RoughlyEqual  slope=0.1
  cmp_2 : UnitTest_Lib/RoughlyEqual  slope=0.1
  cmp_3 : UnitTest_Lib/RoughlyEqual  slope=0.1
  result_tws : ToWorkspace  VariableName=spec_result_005
  tws_1 : ToWorkspace  VariableName=spec_req_005_001
  tws_2 : ToWorkspace  VariableName=spec_req_005_002
  tws_3 : ToWorkspace  VariableName=spec_req_005_003
  result : Outport
  wires:
  sig_Req_Bus/1 -> BS_Req/1
  sig_Result_Bus/1 -> BS_Result/1
  AndN/1 -> result/1, result_tws/1
  BS_Req/1 -> cmp_1/1, Scope1/1  "<testSig_BattU_u>"
  BS_Result/1 -> cmp_1/2, Scope1/2  "<BattU_u>"
  cmp_1/1 -> Bitwise_And1/1
  Bitwise_And1/1 -> tws_1/1, AndN/1, Scope/1
  BS_Req/2 -> cmp_2/1, Scope2/1  "<testSig_BattU_facCor>"
  BS_Result/2 -> cmp_2/2, Scope2/2  "<BattU_facCor>"
  cmp_2/1 -> Bitwise_And2/1
  Bitwise_And2/1 -> tws_2/1, AndN/2, Scope/2
  BS_Req/3 -> cmp_3/1, Scope3/1  "<testSig_BattU_uRated>"
  BS_Result/3 -> cmp_3/2, Scope3/2  "<BattU_uRated>"
  cmp_3/1 -> Bitwise_And3/1
  Bitwise_And3/1 -> tws_3/1, AndN/3, Scope/3
